simulink library "Collector_1xN"  (R2018b)
settings: Solver=ode45  StartTime=0.0  StopTime=10.0  RelTol=1e-3  EnableMultiTasking=on
libraries: carnot x4
settings Model: Creator=lena.frank  LastModifiedBy=drhf
settings DataIOCC: LimitDataPoints=on  SaveFormat=Array  SignalLoggingSaveFormat=ModelDataLogs
settings OptimizationCC: ExpressionDepthLimit=2147483647  LifeSpan=inf
settings DebuggingCC: UnderspecifiedInitializationDetection=Classic  MergeDetectMultiDrivingBlocksExec=none  SolverPrmCheckMsg=warning  FcnCallInpInsideContextMsg=warning  StateNameClashWarn=warning  SFUnexpectedBacktrackingDiag=warning  SFNoUnconditionalDefaultTransitionDiag=warning  SFExecutionAtInitializationDiag=none
settings HardwareCC: ProdBitPerPointer=32  ProdBitPerSizeT=32  ProdBitPerPtrDiffT=32  ProdLargestAtomicFloat=None  ProdIntDivRoundTo=Undefined  ProdEndianess=Unspecified  ProdWordSize=32  ProdHWDeviceType=32-bit Generic
settings ModelReferenceCC: PropagateSignalLabelsOutOfModel=off
settings SFSimCC: SimUseLocalCustomCode=off
settings RTWCC: RTWUseLocalCustomCode=off
settings CodeAppCC: StateflowObjectComments=on
settings GRTTargetCC: TargetLangStandard=C89/C90 (ANSI)  GeneratePreprocessorConditionals=Disable all  CombineOutputUpdateFcns=off  GRTInterface=on
settings ConfigComp: CovMetricSettings=dw  CovHtmlReporting=on  CovSaveCumulativeToWorkspaceVar=on  CovSaveSingleToWorkspaceVar=on  CovExternalEMLEnable=off

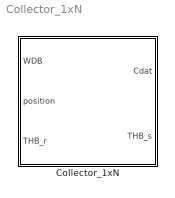
== system Collector_1xN ==
  Collector_1xN : Subsystem  mask(collector 1xN){acol=2.3, len=2, eta0=0.8, u1=3.5, u2=0.02, u3=0, uwind=0, c_col=1e4, lin=10, qua=10, tini=20, nodes=5}
      mask prompts: acol "collector surface (aperture) in [m²]"; len "length between inlet and outlet [m]"; eta0 "optical efficiency [-]"; u1 "linear heat loss coefficient [W/(m²*K)]"; u2 "quadratic heat loss coefficient [W/(m*K)²]"; u3 "radiative loss coefficient [W/(m²*K)]"; uwind "wind dependent heat loss [W/(m²*K*m/s)]"; c_col "effective heat capacity of collector [J/(m²*K)]"; lin "linear pressure drop Pa/(kg/s)"; qua "quadratic  pressure drop Pa/(kg/s)²"; tini "initial temperature [degree Celsius]"; nodes "number of nodes"
      mask help:
      | Model for tested collectors. Enter test results in this mask.
      | Look under mask to change the incidence angle modifier, the pressure drop and the radiation calculation method.
      mask init:
      | acol = max(acol, 0.01);
      | eta0 = max(eta0,0);
      | c_col = max(c_col, 0.1);
      mask Help: web(fullfile(path_carnot('help'),'Collector_1xN.html'),'-helpbrowser')
      mask DialogControl ParameterTabVar0 Prompt: Geometry
      mask DialogControl ParameterTabVar01 Prompt: Coll.Parameters
      mask DialogControl ParameterTabVar012 Prompt: Hydraulic
      mask DialogControl ParameterTabVar0123 Prompt: Calculation
      mask Display: plot(-10,0,80,78,[10 16 66 60 10],[16 10 60 66 16],[8,13],[8,13],[63,68],[63,68])

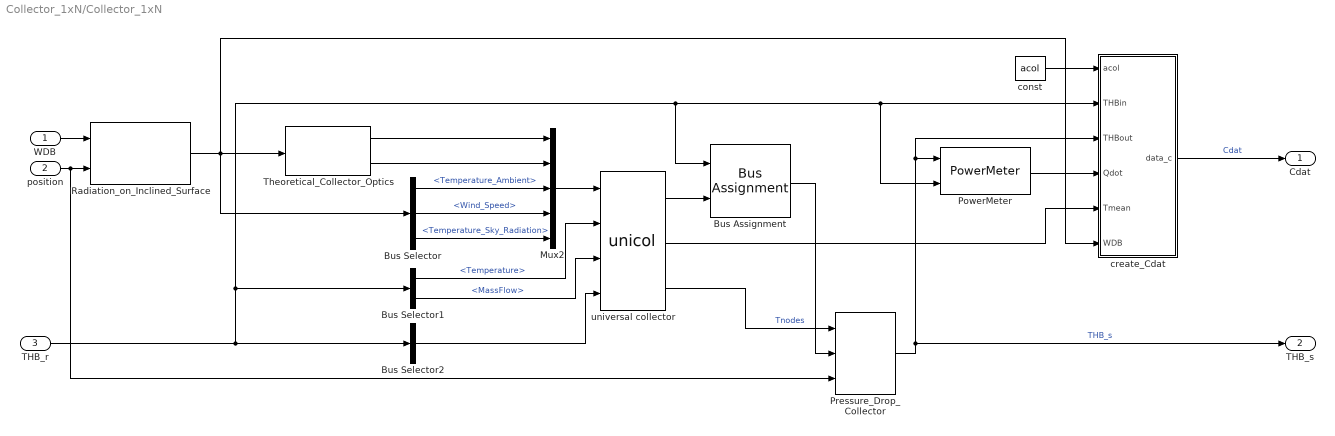
== system Collector_1xN/Collector_1xN ==
  WDB : Inport
  position : Inport  Port=2
  THB_r : Inport  Port=3
  Bus Assignment : BusAssignment  AssignedSignals=Temperature
  Bus Selector : BusSelector  OutputSignals=Temperature_Ambient,Wind_Speed,Temperature_Sky_Radiation
  Bus Selector1 : BusSelector  OutputSignals=Temperature,MassFlow
  Bus Selector2 : BusSelector  OutputSignals=Pressure,FluidType,FluidMix  OutputAsBus=on
  Mux2 : Mux  Inputs=5
  PowerMeter : carnot/Control/PowerMeter
      settings: SourceProductName=Carnot
  Pressure_Drop_Collector : carnot/Basic/Pressure_Drop/Pressure_Drop_Collector  len=len  lin=lin  qua=qua
      settings: SourceProductName=Carnot
  Radiation_on_Inclined_Surface : carnot/Weather/Radiation_on_Inclined_Surface  sky=Perez 1990  reflect=0.2
      settings: SourceProductName=Carnot
  Theoretical_Collector_Optics : carnot/Source/Solar_Thermal/IncidenceAngleModifier/Theoretical_Collector_Optics  FTA=eta0  ncover=1  refin=1.525  d=0.004  ext=4
      settings: SourceProductName=Carnot
  const : Constant  Value=acol
  create_Cdat : Subsystem
  universal collector : S-Function  FunctionName=unicol  Parameters=acol, u1, u2, u3, uwind, c_col, tini, nodes  SFunctionDeploymentMode=off  EnableBusSupport=off
  Cdat : Outport
  THB_s : Outport  Port=2
  wires:
  create_Cdat/1(data_c) -> Cdat/1  "Cdat"
  const/1 -> create_Cdat/1(acol)
  THB_r/1 -> Bus Selector1/1, Bus Assignment/1, create_Cdat/2(THBin), PowerMeter/2, Bus Selector2/1
  WDB/1 -> Radiation_on_Inclined_Surface/1
  position/1 -> Radiation_on_Inclined_Surface/2, Pressure_Drop_Collector/3
  Radiation_on_Inclined_Surface/1 -> create_Cdat/6(WDB), Theoretical_Collector_Optics/1, Bus Selector/1
  universal collector/2 -> create_Cdat/5(Tmean)
  universal collector/1 -> Bus Assignment/2
  Pressure_Drop_Collector/1 -> THB_s/1, create_Cdat/3(THBout), PowerMeter/1  "THB_s"
  Bus Selector/2 -> Mux2/4  "<Wind_Speed>"
  Bus Selector/1 -> Mux2/3  "<Temperature_Ambient>"
  Theoretical_Collector_Optics/1 -> Mux2/1
  Theoretical_Collector_Optics/2 -> Mux2/2
  Bus Selector/3 -> Mux2/5  "<Temperature_Sky_Radiation>"
  Mux2/1 -> universal collector/1
  Bus Selector1/1 -> universal collector/2  "<Temperature>"
  Bus Selector1/2 -> universal collector/3  "<MassFlow>"
  Bus Selector2/1 -> universal collector/4
  PowerMeter/1 -> create_Cdat/4(Qdot)
  universal collector/3 -> Pressure_Drop_Collector/1  "Tnodes"
  Bus Assignment/1 -> Pressure_Drop_Collector/2

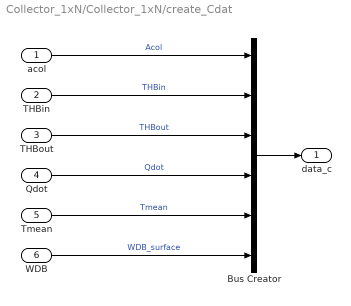
== system Collector_1xN/Collector_1xN/create_Cdat ==
  acol : Inport
  THBin : Inport  Port=2
  THBout : Inport  Port=3
  Qdot : Inport  Port=4
  Tmean : Inport  Port=5
  WDB : Inport  Port=6
  Bus Creator : BusCreator  Inputs=6
  data_c : Outport
  wires:
  acol/1 -> Bus Creator/1  "Acol"
  THBin/1 -> Bus Creator/2  "THBin"
  THBout/1 -> Bus Creator/3  "THBout"
  WDB/1 -> Bus Creator/6  "WDB_surface"
  Bus Creator/1 -> data_c/1
  Qdot/1 -> Bus Creator/4  "Qdot"
  Tmean/1 -> Bus Creator/5  "Tmean"
